simulink model "toy_example"  (R2015b)
settings: Solver=VariableStepAuto  StartTime=0.0  StopTime=10.0  RelTol=1e-3
settings Model: Creator=admin  LastModifiedBy=admin

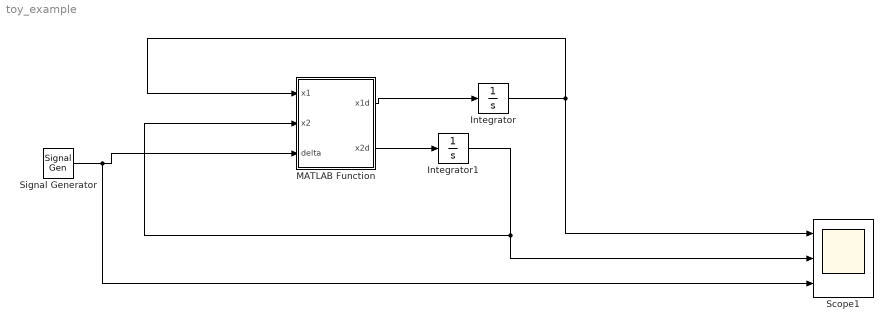
== system toy_example ==
  Integrator : Integrator  InitialCondition=5
  Integrator1 : Integrator  InitialCondition=5
  MATLAB Function : MATLAB Function  TreatAsAtomicUnit=on
  Scope1 : Scope  NumInputPorts=3
  Signal Generator : SignalGenerator  WaveForm=random  Amplitude=10  Units=rad/sec
  wires:
  MATLAB Function/1(x1d) -> Integrator/1
  MATLAB Function/2(x2d) -> Integrator1/1
  Integrator1/1 -> Scope1/2, MATLAB Function/2(x2)
  Integrator/1 -> Scope1/1, MATLAB Function/1(x1)
  Signal Generator/1 -> Scope1/3, MATLAB Function/3(delta)

== matlab function toy_example/MATLAB Function ==
  data: x1 input; x1d output; x2 input; x2d output; delta input
function [x1d,x2d] = fcn(x1,x2,delta)
%#codegen
k1=0.5;
k2=1;
k3=0.5;
x2d=-k1*x1^3;
x2_tilda=x2-x2d;
u=-k2*x2_tilda-x1^3+3*k1*x1^3-3*k1*x1^4*x2-3*k1*k3*x1^4*x2_tilda;
x1d=-x1+x1^2*(x2+delta);
x2d=u;
